simulink model "Winkelsensor"  (R2021b)
settings: Solver=ode3  StartTime=0.0  StopTime=10.0  FixedStep=0.01  RelTol=1e-3
settings Model: Creator=mwjae  LastModifiedBy=mwjae

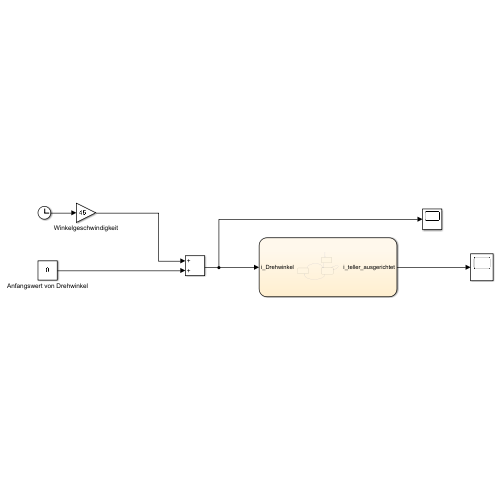
[thumbnail: Simulink's stored preview of the top-level diagram]
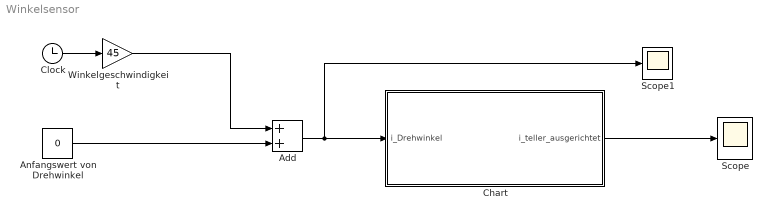
== system Winkelsensor ==
  Add : Sum
  Anfangswert von Drehwinkel : Constant  Value=0
  Chart : Stateflow chart  TreatAsAtomicUnit=on
  Clock : Clock
  Scope : Scope
  Scope1 : Scope
  Winkelgeschwindigkeit : Gain  Gain=45
  wires:
  Clock/1 -> Winkelgeschwindigkeit/1
  Winkelgeschwindigkeit/1 -> Add/1
  Anfangswert von Drehwinkel/1 -> Add/2
  Add/1 -> Scope1/1, Chart/1(i_Drehwinkel)
  Chart/1(i_teller_ausgerichtet) -> Scope/1

== stateflow chart Winkelsensor/Chart ==
  state start
  state Ausgerichtet
    i_teller_ausgerichtet = 1;
  state nichtAusgerichtet
    i_teller_ausgerichtet = 0;
  (default) -> start
  start -> Ausgerichtet : [i_Drehwinkel>=88]
  nichtAusgerichtet -> Ausgerichtet : [(0<=mod(i_Drehwinkel,90)&mod(i_Drehwinkel,90)<=2)|(88<=mod(i_Drehwinkel,90)&mod(i_Drehwinkel,90)<90)]
  Ausgerichtet -> Ausgerichtet [order 1] : [(0<=mod(i_Drehwinkel,90)&mod(i_Drehwinkel,90)<=2)|(88<=mod(i_Drehwinkel,90)&mod(i_Drehwinkel,90)<90)]
  Ausgerichtet -> nichtAusgerichtet [order 2] : [(mod(i_Drehwinkel,90)>2 & (mod(i_Drehwinkel,90)<88)|89<mod(i_Drehwinkel,90))]
  data: i_Drehwinkel input; i_teller_ausgerichtet output
